simulink model "untitled"  (R2013a)
settings: Solver=ode45  StartTime=0.0  StopTime=70.0  RelTol=1e-6
settings Model: Creator=David  LastModifiedBy=David

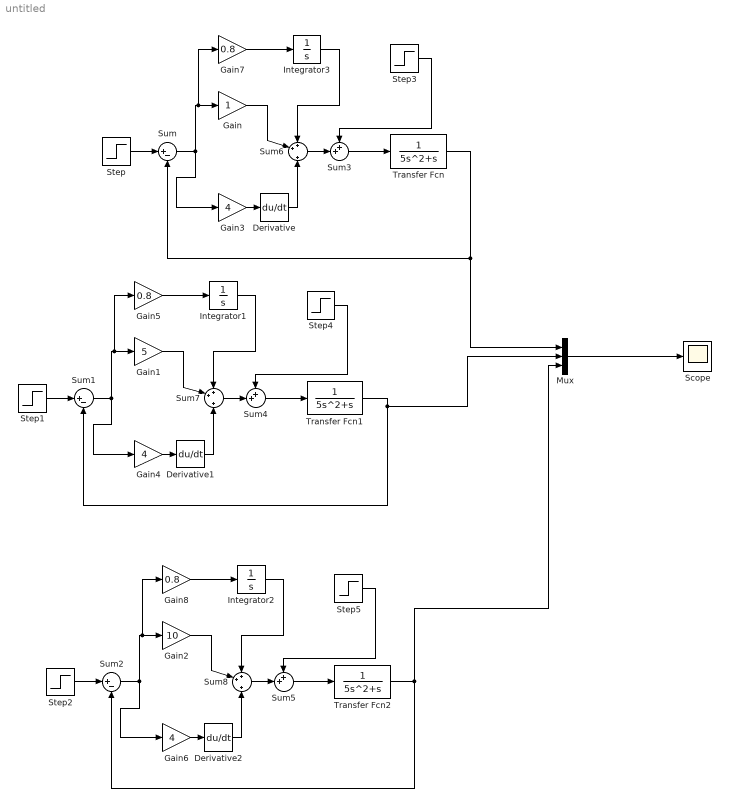
== system untitled ==
  Derivative : Derivative
  Derivative1 : Derivative
  Derivative2 : Derivative
  Gain : Gain
  Gain1 : Gain  Gain=5
  Gain2 : Gain  Gain=10
  Gain3 : Gain  Gain=4
  Gain4 : Gain  Gain=4
  Gain5 : Gain  Gain=0.8
  Gain6 : Gain  Gain=4
  Gain7 : Gain  Gain=0.8
  Gain8 : Gain  Gain=0.8
  Integrator1 : Integrator
  Integrator2 : Integrator
  Integrator3 : Integrator
  Mux : Mux  Inputs=3
  Scope : Scope
  Step : Step  SampleTime=0
  Step1 : Step  SampleTime=0
  Step2 : Step  SampleTime=0
  Step3 : Step  Time=60  After=-0.3  SampleTime=0
  Step4 : Step  Time=60  After=-0.3  SampleTime=0
  Step5 : Step  Time=60  After=-0.3  SampleTime=0
  Sum : Sum  Inputs=|+-
  Sum1 : Sum  Inputs=|+-
  Sum2 : Sum  Inputs=|+-
  Sum3 : Sum  Inputs=++|
  Sum4 : Sum  Inputs=++|
  Sum5 : Sum  Inputs=++|
  Sum6 : Sum  Inputs=++|+
  Sum7 : Sum  Inputs=++|+
  Sum8 : Sum  Inputs=++|+
  Transfer Fcn : TransferFcn  Denominator=[5 1 0]
  Transfer Fcn1 : TransferFcn  Denominator=[5 1 0]
  Transfer Fcn2 : TransferFcn  Denominator=[5 1 0]
  wires:
  Step/1 -> Sum/1
  Sum3/1 -> Transfer Fcn/1
  Step3/1 -> Sum3/1
  Sum/1 -> Gain3/1, Gain7/1, Gain/1
  Sum6/1 -> Sum3/2
  Gain3/1 -> Derivative/1
  Transfer Fcn/1 -> Mux/1, Sum/2
  Derivative/1 -> Sum6/3
  Gain/1 -> Sum6/2
  Integrator3/1 -> Sum6/1
  Gain7/1 -> Integrator3/1
  Step1/1 -> Sum1/1
  Sum4/1 -> Transfer Fcn1/1
  Step4/1 -> Sum4/1
  Sum1/1 -> Gain4/1, Gain5/1, Gain1/1
  Sum7/1 -> Sum4/2
  Gain4/1 -> Derivative1/1
  Derivative1/1 -> Sum7/3
  Gain1/1 -> Sum7/2
  Integrator1/1 -> Sum7/1
  Gain5/1 -> Integrator1/1
  Transfer Fcn1/1 -> Mux/2, Sum1/2
  Step2/1 -> Sum2/1
  Sum5/1 -> Transfer Fcn2/1
  Step5/1 -> Sum5/1
  Sum2/1 -> Gain6/1, Gain8/1, Gain2/1
  Sum8/1 -> Sum5/2
  Gain6/1 -> Derivative2/1
  Derivative2/1 -> Sum8/3
  Gain2/1 -> Sum8/2
  Integrator2/1 -> Sum8/1
  Gain8/1 -> Integrator2/1
  Transfer Fcn2/1 -> Mux/3, Sum2/2
  Mux/1 -> Scope/1
